simulink model "main"  (R2021b)
settings: Solver=VariableStepAuto  StartTime=0.0  StopTime=100  MaxStep=1e-3  RelTol=1e-4
settings Model: Creator=Pietro  LastModifiedBy=anand

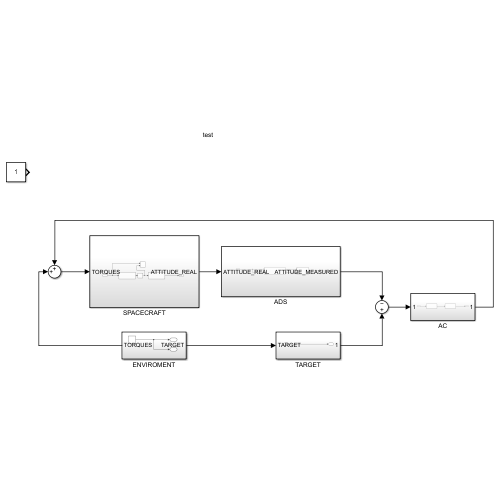
[thumbnail: Simulink's stored preview of the top-level diagram]
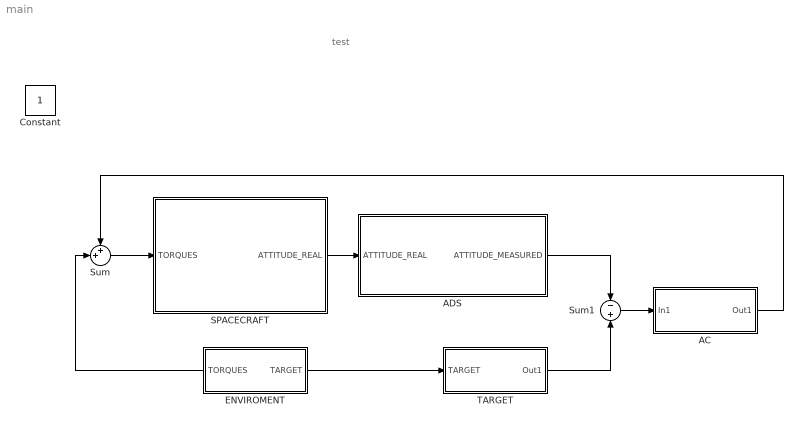
== system main ==
  note: test
  AC : Subsystem
  ADS : Subsystem
  Constant : Constant
  ENVIROMENT : Subsystem
      settings: PortSchema="{\"entries\":[{\"content\":{\"sides\":[{\"content\":{\"connectorIds\":[\"Out2\"]},\"type\":\"ConnectorPlacement.EquallySpacedRectSide\",\"uuid\":\"3513c087-c4e3-49ca-8f09-1f9f820f004f\"},{\"content\":{\"connectorIds\":[\"Out1\"],\"side\":\"RIGHT\"},\"type\":\"ConnectorPlacement.EquallySpacedRectSide\",\"uuid\":\"ea215f41-dce9-47b1-a5af-17461ae57bf5\"},{\"content\":{\"connectorIds\":[],\"side\":\"TOP\"},\"type\":\"ConnectorPlacement.EquallySpacedRectSide\",\"uuid\":\"191a9640-43fb-47cb-a633-1e69fb686a5c\"}]},\"type\":\"ConnectorPlacement.EquallySpacedConnector\",\"uuid\":\"76c74810-6da4-4e68-9ef1-4b58edbbd43a\"}],\"packageUris\":[\"http://schema.mathworks.com/mf0/Connector/R2020b\"],\"version\":\"1.0\"}"
  SPACECRAFT : Subsystem
  Sum : Sum  Inputs=++|
  Sum1 : Sum  Inputs=-|+
  TARGET : Subsystem
  wires:
  SPACECRAFT/1(ATTITUDE_REAL) -> ADS/1(ATTITUDE_REAL)
  Sum/1 -> SPACECRAFT/1(TORQUES)
  AC/1(Out1) -> Sum/1
  TARGET/1(Out1) -> Sum1/2
  ADS/1(ATTITUDE_MEASURED) -> Sum1/1
  Sum1/1 -> AC/1(In1)
  ENVIROMENT/1(TARGET) -> TARGET/1(TARGET)
  ENVIROMENT/2(TORQUES) -> Sum/2

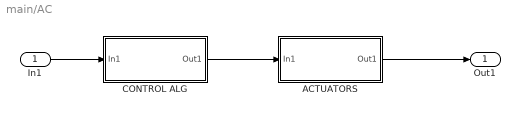
== system main/AC ==
  In1 : Inport
  ACTUATORS : Subsystem
  CONTROL ALG : Subsystem
  Out1 : Outport
  wires:
  CONTROL ALG/1(Out1) -> ACTUATORS/1(In1)
  In1/1 -> CONTROL ALG/1(In1)
  ACTUATORS/1(Out1) -> Out1/1

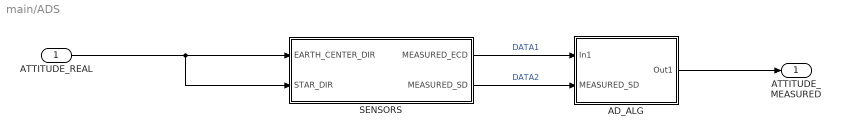
== system main/ADS ==
  ATTITUDE_REAL : Inport
  AD_ALG : Subsystem
  SENSORS : Subsystem
  ATTITUDE_MEASURED : Outport
  wires:
  ATTITUDE_REAL/1 -> SENSORS/2(STAR_DIR), SENSORS/1(EARTH_CENTER_DIR)
  AD_ALG/1(Out1) -> ATTITUDE_MEASURED/1
  SENSORS/1(MEASURED_ECD) -> AD_ALG/1(In1)  "DATA1"
  SENSORS/2(MEASURED_SD) -> AD_ALG/2(MEASURED_SD)  "DATA2"

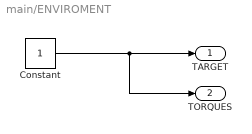
== system main/ENVIROMENT ==
  Constant : Constant
  TARGET : Outport
  TORQUES : Outport  Port=2
  wires:
  Constant/1 -> TORQUES/1, TARGET/1

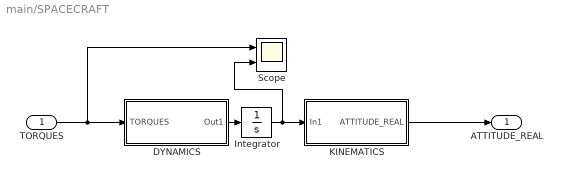
== system main/SPACECRAFT ==
  TORQUES : Inport
  DYNAMICS : Subsystem
  Integrator : Integrator  InitialCondition=1
  KINEMATICS : Subsystem
  Scope : Scope  NumInputPorts=2
  ATTITUDE_REAL : Outport
  wires:
  DYNAMICS/1(Out1) -> Integrator/1
  KINEMATICS/1(ATTITUDE_REAL) -> ATTITUDE_REAL/1
  TORQUES/1 -> Scope/1, DYNAMICS/1(TORQUES)
  Integrator/1 -> Scope/2, KINEMATICS/1(In1)

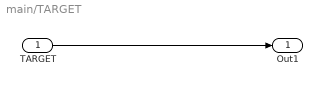
== system main/TARGET ==
  TARGET : Inport
  Out1 : Outport
  wires:
  TARGET/1 -> Out1/1

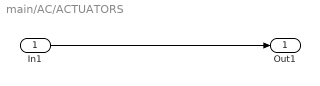
== system main/AC/ACTUATORS ==
  In1 : Inport
  Out1 : Outport
  wires:
  In1/1 -> Out1/1

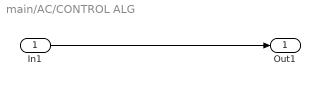
== system main/AC/CONTROL ALG ==
  In1 : Inport
  Out1 : Outport
  wires:
  In1/1 -> Out1/1

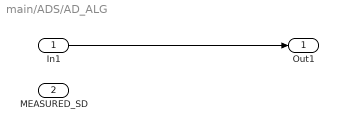
== system main/ADS/AD_ALG ==
  In1 : Inport
  MEASURED_SD : Inport  Port=2
  Out1 : Outport
  wires:
  In1/1 -> Out1/1

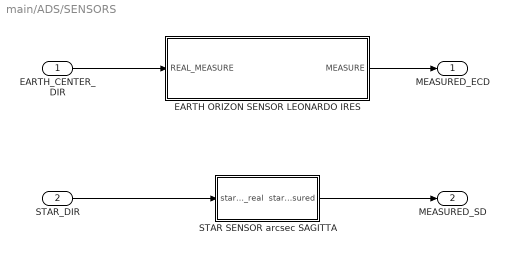
== system main/ADS/SENSORS ==
  EARTH_CENTER_DIR : Inport
  STAR_DIR : Inport  Port=2
  EARTH ORIZON SENSOR LEONARDO IRES : Subsystem
  STAR SENSOR arcsec SAGITTA : Subsystem
  MEASURED_ECD : Outport
  MEASURED_SD : Outport  Port=2
  wires:
  EARTH ORIZON SENSOR LEONARDO IRES/1(MEASURE) -> MEASURED_ECD/1
  EARTH_CENTER_DIR/1 -> EARTH ORIZON SENSOR LEONARDO IRES/1(REAL_MEASURE)
  STAR_DIR/1 -> STAR SENSOR arcsec SAGITTA/1(star_vector_real)
  STAR SENSOR arcsec SAGITTA/1(star_versor_measured) -> MEASURED_SD/1

== system main/SPACECRAFT/DYNAMICS ==
  TORQUES : Inport
  Out1 : Outport
  wires:
  TORQUES/1 -> Out1/1

== system main/SPACECRAFT/KINEMATICS ==
  In1 : Inport
  ATTITUDE_REAL : Outport
  wires:
  In1/1 -> ATTITUDE_REAL/1

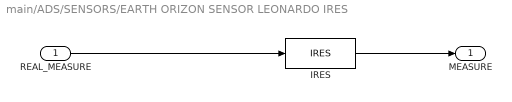
== system main/ADS/SENSORS/EARTH ORIZON SENSOR LEONARDO IRES ==
  REAL_MEASURE : Inport
  IRES : MATLABFcn  MATLABFcn=IRES
  MEASURE : Outport
  wires:
  IRES/1 -> MEASURE/1
  REAL_MEASURE/1 -> IRES/1

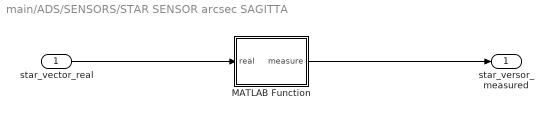
== system main/ADS/SENSORS/STAR SENSOR arcsec SAGITTA ==
  star_vector_real : Inport
  MATLAB Function : MATLAB Function  TreatAsAtomicUnit=on
  star_versor_measured : Outport
  wires:
  star_vector_real/1 -> MATLAB Function/1(real)
  MATLAB Function/1(measure) -> star_versor_measured/1

== matlab function main/ADS/SENSORS/STAR SENSOR arcsec SAGITTA/MATLAB Function ==
  data: real input; measure output
function measure = SAGITTA(real)
    %Author: Pietro Spinelli
    %arcsec SAGITTA Star Tracker:
    %<https://www.cubesatshop.com/product/kul-star-tracker/>
    
    
    acc_b=10/3600;      %Boresight accuracy [deg]
    acc_o=2/3600;       %Cross accuracy [deg]
    
    angle_cross1=random('Normal',0,acc_o); %Rotation error x [deg]
    angle_cross2=random('Normal',0,acc_o); %Rotation error y [deg]
    angle_bore=random('Normal',0,acc_b);   %Rotation error z [deg]
     
    
    err_mat=[1 angle_bore -angle_cross1;-angle_bore 1 angle_cross2; angle_cross2 -angle_cross1 1]; %Error matrix
    measure = err_mat*real; %Real star direction gets rotated by error matrix




end
